simulink model "NonisothermalCSTR_closedLoop"  (R2024a)
settings: Solver=ode23s  StartTime=0.0  StopTime=3600*4  RelTol=1e-3
undefined symbols (not defined in the file): u_simulate
libraries: slpidlib x3
settings Model: Creator=tmlouw  LastModifiedBy=tmlouw

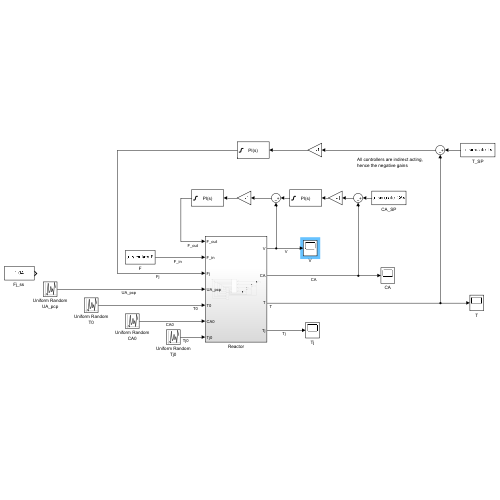
[thumbnail: Simulink's stored preview of the top-level diagram]
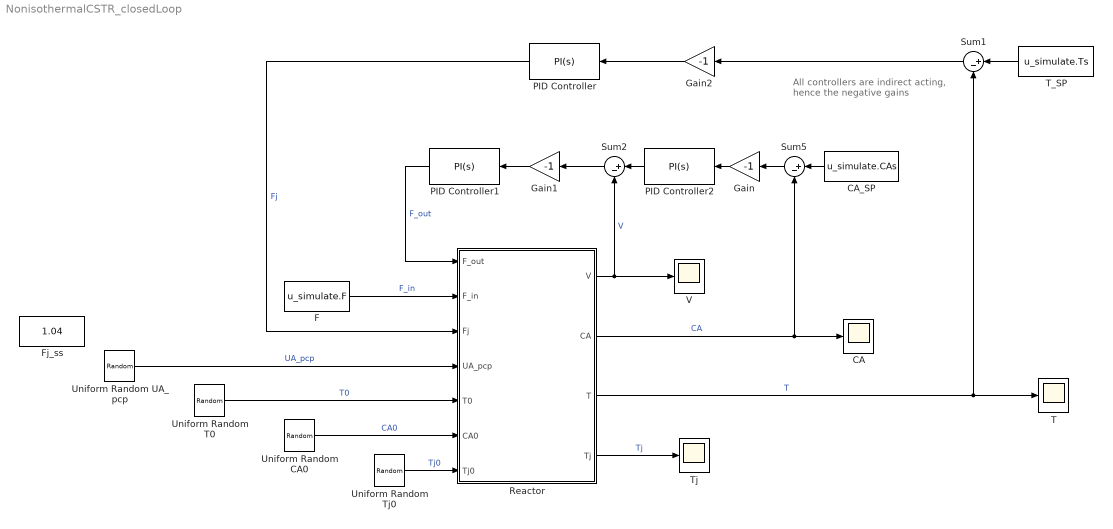
== system NonisothermalCSTR_closedLoop ==
  note: All controllers are indirect acting, hence the negative gains
  CA : Scope
  CA_SP : Constant  Value=u_simulate.CAs
  F : Constant  Value=u_simulate.F
  "Fj_ss " : Constant  Value=1.04
  Gain : Gain  Gain=-1
  Gain1 : Gain  Gain=-1
  Gain2 : Gain  Gain=-1
  PID Controller : slpidlib/PID Controller  Controller=PI  Form=Parallel  TimeDomain=Continuous-time  UseExternalTs=off  SampleTime=-1  IntegratorMethod=Forward Euler  FilterMethod=Forward Euler  ControllerParametersSource=internal  P=10  I=0  UseKiTs=off  D=0  UseExternalDerivativeSource=off  N=100  UseFilter=on  TunerSelectOption=Transfer Function Based (PID Tuner App)  InitialConditionSource=internal  InitialConditionForIntegrator=1.04  InitialConditionForFilter=0  DifferentiatorICPrevScaledInput=0  ExternalReset=none  TrackingMode=off  Kt=1  LimitOutput=on  SatLimitsSource=internal  UpperSaturationLimit=5  LowerSaturationLimit=0  LinearizeAsGain=on  AntiWindupMode=clamping  Kb=1  LimitIntegrator=off  UpperIntegratorSaturationLimit=inf  LowerIntegratorSaturationLimit=-inf  POutMin=[]  POutMax=[]  IOutMin=[]  IOutMax=[]  DOutMin=[]  DOutMax=[]  NOutMin=[]  NOutMax=[]  SumOutMin=[]  SumOutMax=[]  SaturationOutMin=[]  SaturationOutMax=[]  PParamMin=[]  PParamMax=[]  IParamMin=[]  IParamMax=[]  DParamMin=[]  DParamMax=[]  NParamMin=[]  NParamMax=[]  KbParamMin=[]  KbParamMax=[]  KtParamMin=[]  KtParamMax=[]  KbOutMin=[]  KbOutMax=[]  KtOutMin=[]  KtOutMax=[]  IntegratorOutMin=[]  IntegratorOutMax=[]  FilterOutMin=[]  FilterOutMax=[]  SumI1OutMin=[]  SumI1OutMax=[]  SumI2OutMin=[]  SumI2OutMax=[]  SumI3OutMin=[]  SumI3OutMax=[]  SumI4OutMin=[]  SumI4OutMax=[]  SumDOutMin=[]  SumDOutMax=[]  DifferentiatorOutMin=[]  DifferentiatorOutMax=[]  FilterDiffOutCoefMin=[]  FilterDiffOutCoefMax=[]  ReciprocalOutMin=[]  ReciprocalOutMax=[]  SumDenOutMin=[]  SumDenOutMax=[]  SumNumOutMin=[]  SumNumOutMax=[]  DivideOutMin=[]  DivideOutMax=[]  UdiffTsProdOutMin=[]  UdiffTsProdOutMax=[]  NTsProdOutMin=[]  NTsProdOutMax=[]  UintegralTsProdOutMin=[]  UintegralTsProdOutMax=[]  UngainTsProdOutMin=[]  UngainTsProdOutMax=[]  ClampingZeroOutDataTypeStr=Inherit: Inherit via back propagation  ClampingZeroOutMin=[]  ClampingZeroOutMax=[]  FilterDenConstantOutDataTypeStr=Inherit: Inherit via back propagation  FilterDenConstantOutMin=[]  FilterDenConstantOutMax=[]  PCopyOutDataTypeStr=Inherit: Inherit via back propagation  PCopyOutMin=[]  PCopyOutMax=[]  NCopyOutDataTypeStr=Inherit: Inherit via back propagation  NCopyOutMin=[]  NCopyOutMax=[]  IntegratorContinuousStateAttributes=''  IntegratorStateMustResolveToSignalObject=off  IntegratorRTWStateStorageClass=Auto  FilterContinuousStateAttributes=''  FilterStateMustResolveToSignalObject=off  FilterRTWStateStorageClass=Auto  ParallelPVariant=InternalParameters  IdealPVariant=Disabled  IVariant=InternalParameters  DVariant=Disabled  IntegratorVariant=Continuous  SatVariant=Enabled  AWVariant=ContClampingParallel  PCopyVariant=Disabled  TRVariant=Disabled  FdbkBlocksVariant=Forward  IdealPFdbkVariant=Disabled  SatFdbkVariant=Disabled  DerivativeFilterVariant=Disabled  NVariant=Disabled  NCopyVariant=Disabled_SignalSpec  FilterICVariant=Disabled  IntegratorICVariant=InternalICs  ExternalResetVariant=Disabled  TRSumVariant=Passthrough  SumFdbkVariant=Disabled  SumVariant=Sum_PI  TsampFilterVariant=InternalTs  TsampNgainVariant=Passthrough  TsampIntegralVariant=Disabled_SignalSpec  ExternalSaturationOutDataTypeStr=Inherit: Same as second input  DerivativeSourceVariant=Disabled
  PID Controller1 : slpidlib/PID Controller  Controller=PI  Form=Parallel  TimeDomain=Continuous-time  UseExternalTs=off  SampleTime=-1  IntegratorMethod=Forward Euler  FilterMethod=Forward Euler  ControllerParametersSource=internal  P=50  I=0  UseKiTs=off  D=0  UseExternalDerivativeSource=off  N=100  UseFilter=on  TunerSelectOption=Transfer Function Based (PID Tuner App)  InitialConditionSource=internal  InitialConditionForIntegrator=u_simulate.F  InitialConditionForFilter=0  DifferentiatorICPrevScaledInput=0  ExternalReset=none  TrackingMode=off  Kt=1  LimitOutput=on  SatLimitsSource=internal  UpperSaturationLimit=0.8  LowerSaturationLimit=0.05  LinearizeAsGain=off  AntiWindupMode=none  Kb=1  LimitIntegrator=off  UpperIntegratorSaturationLimit=inf  LowerIntegratorSaturationLimit=-inf  POutMin=[]  POutMax=[]  IOutMin=[]  IOutMax=[]  DOutMin=[]  DOutMax=[]  NOutMin=[]  NOutMax=[]  SumOutMin=[]  SumOutMax=[]  SaturationOutMin=[]  SaturationOutMax=[]  PParamMin=[]  PParamMax=[]  IParamMin=[]  IParamMax=[]  DParamMin=[]  DParamMax=[]  NParamMin=[]  NParamMax=[]  KbParamMin=[]  KbParamMax=[]  KtParamMin=[]  KtParamMax=[]  KbOutMin=[]  KbOutMax=[]  KtOutMin=[]  KtOutMax=[]  IntegratorOutMin=[]  IntegratorOutMax=[]  FilterOutMin=[]  FilterOutMax=[]  SumI1OutMin=[]  SumI1OutMax=[]  SumI2OutMin=[]  SumI2OutMax=[]  SumI3OutMin=[]  SumI3OutMax=[]  SumI4OutMin=[]  SumI4OutMax=[]  SumDOutMin=[]  SumDOutMax=[]  DifferentiatorOutMin=[]  DifferentiatorOutMax=[]  FilterDiffOutCoefMin=[]  FilterDiffOutCoefMax=[]  ReciprocalOutMin=[]  ReciprocalOutMax=[]  SumDenOutMin=[]  SumDenOutMax=[]  SumNumOutMin=[]  SumNumOutMax=[]  DivideOutMin=[]  DivideOutMax=[]  UdiffTsProdOutMin=[]  UdiffTsProdOutMax=[]  NTsProdOutMin=[]  NTsProdOutMax=[]  UintegralTsProdOutMin=[]  UintegralTsProdOutMax=[]  UngainTsProdOutMin=[]  UngainTsProdOutMax=[]  ClampingZeroOutDataTypeStr=Inherit: Inherit via back propagation  ClampingZeroOutMin=[]  ClampingZeroOutMax=[]  FilterDenConstantOutDataTypeStr=Inherit: Inherit via back propagation  FilterDenConstantOutMin=[]  FilterDenConstantOutMax=[]  PCopyOutDataTypeStr=Inherit: Inherit via back propagation  PCopyOutMin=[]  PCopyOutMax=[]  NCopyOutDataTypeStr=Inherit: Inherit via back propagation  NCopyOutMin=[]  NCopyOutMax=[]  IntegratorContinuousStateAttributes=''  IntegratorStateMustResolveToSignalObject=off  IntegratorRTWStateStorageClass=Auto  FilterContinuousStateAttributes=''  FilterStateMustResolveToSignalObject=off  FilterRTWStateStorageClass=Auto  ParallelPVariant=InternalParameters  IdealPVariant=Disabled  IVariant=InternalParameters  DVariant=Disabled  IntegratorVariant=Continuous  SatVariant=Enabled  AWVariant=Passthrough  PCopyVariant=Disabled  TRVariant=Disabled  FdbkBlocksVariant=Forward  IdealPFdbkVariant=Disabled  SatFdbkVariant=Disabled  DerivativeFilterVariant=Disabled  NVariant=Disabled  NCopyVariant=Disabled_SignalSpec  FilterICVariant=Disabled  IntegratorICVariant=InternalICs  ExternalResetVariant=Disabled  TRSumVariant=Passthrough  SumFdbkVariant=Disabled  SumVariant=Sum_PI  TsampFilterVariant=InternalTs  TsampNgainVariant=Passthrough  TsampIntegralVariant=Disabled_SignalSpec  ExternalSaturationOutDataTypeStr=Inherit: Same as second input  DerivativeSourceVariant=Disabled
  PID Controller2 : slpidlib/PID Controller  Controller=PI  Form=Parallel  TimeDomain=Continuous-time  UseExternalTs=off  SampleTime=-1  IntegratorMethod=Forward Euler  FilterMethod=Forward Euler  ControllerParametersSource=internal  P=1000  I=0  UseKiTs=off  D=0  UseExternalDerivativeSource=off  N=100  UseFilter=on  TunerSelectOption=Transfer Function Based (PID Tuner App)  InitialConditionSource=internal  InitialConditionForIntegrator=u_simulate.V  InitialConditionForFilter=0  DifferentiatorICPrevScaledInput=0  ExternalReset=none  TrackingMode=off  Kt=1  LimitOutput=on  SatLimitsSource=internal  UpperSaturationLimit=500  LowerSaturationLimit=100  LinearizeAsGain=on  AntiWindupMode=clamping  Kb=1  LimitIntegrator=off  UpperIntegratorSaturationLimit=inf  LowerIntegratorSaturationLimit=-inf  POutMin=[]  POutMax=[]  IOutMin=[]  IOutMax=[]  DOutMin=[]  DOutMax=[]  NOutMin=[]  NOutMax=[]  SumOutMin=[]  SumOutMax=[]  SaturationOutMin=[]  SaturationOutMax=[]  PParamMin=[]  PParamMax=[]  IParamMin=[]  IParamMax=[]  DParamMin=[]  DParamMax=[]  NParamMin=[]  NParamMax=[]  KbParamMin=[]  KbParamMax=[]  KtParamMin=[]  KtParamMax=[]  KbOutMin=[]  KbOutMax=[]  KtOutMin=[]  KtOutMax=[]  IntegratorOutMin=[]  IntegratorOutMax=[]  FilterOutMin=[]  FilterOutMax=[]  SumI1OutMin=[]  SumI1OutMax=[]  SumI2OutMin=[]  SumI2OutMax=[]  SumI3OutMin=[]  SumI3OutMax=[]  SumI4OutMin=[]  SumI4OutMax=[]  SumDOutMin=[]  SumDOutMax=[]  DifferentiatorOutMin=[]  DifferentiatorOutMax=[]  FilterDiffOutCoefMin=[]  FilterDiffOutCoefMax=[]  ReciprocalOutMin=[]  ReciprocalOutMax=[]  SumDenOutMin=[]  SumDenOutMax=[]  SumNumOutMin=[]  SumNumOutMax=[]  DivideOutMin=[]  DivideOutMax=[]  UdiffTsProdOutMin=[]  UdiffTsProdOutMax=[]  NTsProdOutMin=[]  NTsProdOutMax=[]  UintegralTsProdOutMin=[]  UintegralTsProdOutMax=[]  UngainTsProdOutMin=[]  UngainTsProdOutMax=[]  ClampingZeroOutDataTypeStr=Inherit: Inherit via back propagation  ClampingZeroOutMin=[]  ClampingZeroOutMax=[]  FilterDenConstantOutDataTypeStr=Inherit: Inherit via back propagation  FilterDenConstantOutMin=[]  FilterDenConstantOutMax=[]  PCopyOutDataTypeStr=Inherit: Inherit via back propagation  PCopyOutMin=[]  PCopyOutMax=[]  NCopyOutDataTypeStr=Inherit: Inherit via back propagation  NCopyOutMin=[]  NCopyOutMax=[]  IntegratorContinuousStateAttributes=''  IntegratorStateMustResolveToSignalObject=off  IntegratorRTWStateStorageClass=Auto  FilterContinuousStateAttributes=''  FilterStateMustResolveToSignalObject=off  FilterRTWStateStorageClass=Auto  ParallelPVariant=InternalParameters  IdealPVariant=Disabled  IVariant=InternalParameters  DVariant=Disabled  IntegratorVariant=Continuous  SatVariant=Enabled  AWVariant=ContClampingParallel  PCopyVariant=Disabled  TRVariant=Disabled  FdbkBlocksVariant=Forward  IdealPFdbkVariant=Disabled  SatFdbkVariant=Disabled  DerivativeFilterVariant=Disabled  NVariant=Disabled  NCopyVariant=Disabled_SignalSpec  FilterICVariant=Disabled  IntegratorICVariant=InternalICs  ExternalResetVariant=Disabled  TRSumVariant=Passthrough  SumFdbkVariant=Disabled  SumVariant=Sum_PI  TsampFilterVariant=InternalTs  TsampNgainVariant=Passthrough  TsampIntegralVariant=Disabled_SignalSpec  ExternalSaturationOutDataTypeStr=Inherit: Same as second input  DerivativeSourceVariant=Disabled
  Reactor : Subsystem
  Sum1 : Sum  Inputs=|+-
  Sum2 : Sum  Inputs=|+-
  Sum5 : Sum  Inputs=|+-
  T : Scope
  T_SP : Constant  Value=u_simulate.Ts
  Tj : Scope
  Uniform Random CA0 : UniformRandomNumber  Minimum=19  Maximum=21  Seed=1  SampleTime=200
  Uniform Random T0 : UniformRandomNumber  Minimum=295  Maximum=305  Seed=2  SampleTime=200
  Uniform Random Tj0 : UniformRandomNumber  Minimum=278  Maximum=288  SampleTime=200
  Uniform Random UA_pcp : UniformRandomNumber  Minimum=0.33  Maximum=0.37  Seed=3  SampleTime=500
  V : Scope
  wires:
  Uniform Random UA_pcp/1 -> Reactor/4(UA_pcp)  "UA_pcp"
  Uniform Random T0/1 -> Reactor/5(T0)  "T0"
  Uniform Random CA0/1 -> Reactor/6(CA0)  "CA0"
  Reactor/1(V) -> V/1, Sum2/2  "V"
  Reactor/2(CA) -> Sum5/2, CA/1  "CA"
  Reactor/3(T) -> Sum1/2, T/1  "T"
  Reactor/4(Tj) -> Tj/1  "Tj"
  F/1 -> Reactor/2(F_in)  "F_in"
  PID Controller/1 -> Reactor/3(Fj)  "Fj"
  T_SP/1 -> Sum1/1
  Sum1/1 -> Gain2/1
  Sum2/1 -> Gain1/1
  PID Controller1/1 -> Reactor/1(F_out)  "F_out"
  PID Controller2/1 -> Sum2/1
  CA_SP/1 -> Sum5/1
  Sum5/1 -> Gain/1
  Uniform Random Tj0/1 -> Reactor/7(Tj0)  "Tj0"
  Gain/1 -> PID Controller2/1
  Gain1/1 -> PID Controller1/1
  Gain2/1 -> PID Controller/1

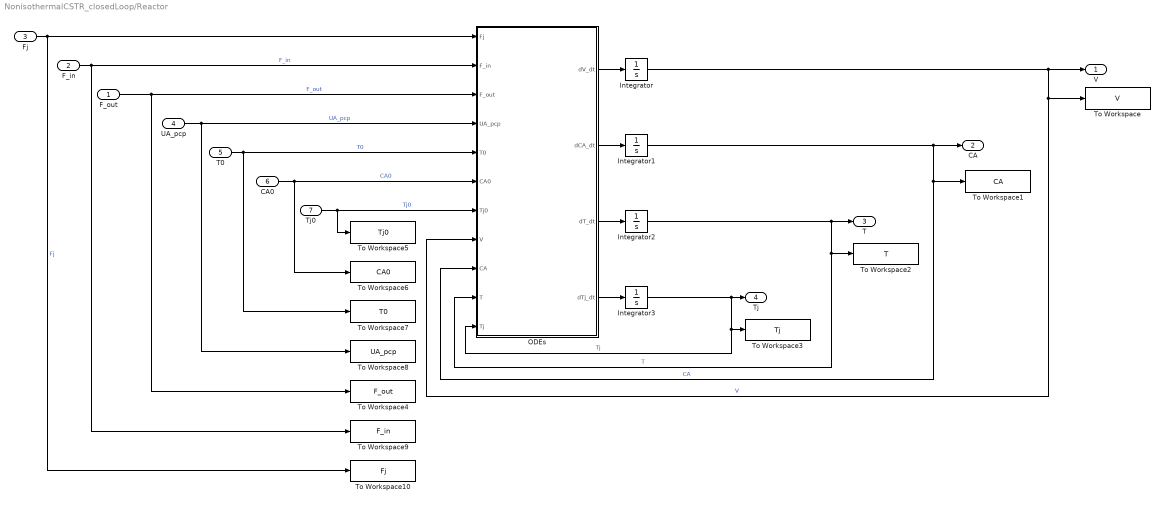
== system NonisothermalCSTR_closedLoop/Reactor ==
  F_out : Inport
  F_in : Inport  Port=2
  Fj : Inport  Port=3
  UA_pcp : Inport  Port=4
  T0 : Inport  Port=5
  CA0 : Inport  Port=6
  Tj0 : Inport  Port=7
  Integrator : Integrator  InitialCondition=u_simulate.V
  Integrator1 : Integrator  InitialCondition=u_simulate.CAs
  Integrator2 : Integrator  InitialCondition=u_simulate.Ts
  Integrator3 : Integrator  InitialCondition=u_simulate.Tjs
  ODEs : MATLAB Function  TreatAsAtomicUnit=on
  To Workspace : ToWorkspace  VariableName=V  SampleTime=1
  To Workspace1 : ToWorkspace  VariableName=CA  SampleTime=1
  To Workspace10 : ToWorkspace  VariableName=Fj  SampleTime=1
  To Workspace2 : ToWorkspace  VariableName=T  SampleTime=1
  To Workspace3 : ToWorkspace  VariableName=Tj  SampleTime=1
  To Workspace4 : ToWorkspace  VariableName=F_out  SampleTime=1
  To Workspace5 : ToWorkspace  VariableName=Tj0  SampleTime=1
  To Workspace6 : ToWorkspace  VariableName=CA0  SampleTime=1
  To Workspace7 : ToWorkspace  VariableName=T0  SampleTime=1
  To Workspace8 : ToWorkspace  VariableName=UA_pcp  SampleTime=1
  To Workspace9 : ToWorkspace  VariableName=F_in  SampleTime=1
  V : Outport
  CA : Outport  Port=2
  T : Outport  Port=3
  Tj : Outport  Port=4
  wires:
  Integrator3/1 -> ODEs/11(Tj), To Workspace3/1, Tj/1  "Tj"
  Integrator2/1 -> T/1, To Workspace2/1, ODEs/10(T)  "T"
  ODEs/1(dV_dt) -> Integrator/1
  ODEs/2(dCA_dt) -> Integrator1/1
  Integrator/1 -> V/1, To Workspace/1, ODEs/8(V)  "V"
  ODEs/3(dT_dt) -> Integrator2/1
  ODEs/4(dTj_dt) -> Integrator3/1
  F_in/1 -> To Workspace9/1, ODEs/2(F_in)  "F_in"
  T0/1 -> ODEs/5(T0), To Workspace7/1  "T0"
  UA_pcp/1 -> To Workspace8/1, ODEs/4(UA_pcp)  "UA_pcp"
  CA0/1 -> To Workspace6/1, ODEs/6(CA0)  "CA0"
  F_out/1 -> ODEs/3(F_out), To Workspace4/1  "F_out"
  Tj0/1 -> ODEs/7(Tj0), To Workspace5/1  "Tj0"
  Integrator1/1 -> CA/1, To Workspace1/1, ODEs/9(CA)  "CA"
  Fj/1 -> To Workspace10/1, ODEs/1(Fj)  "Fj"

== matlab function NonisothermalCSTR_closedLoop/Reactor/ODEs ==
  data: Fj input; F_in input; F_out input; UA_pcp input; T0 input; CA0 input; Tj0 input; V input; CA input; T input; Tj input; dV_dt output; dCA_dt output; dT_dt output; dTj_dt output
function [dV_dt, dCA_dt, dT_dt, dTj_dt] = ODEs(Fj, F_in, F_out, UA_pcp, T0, CA0, Tj0, V, CA, T, Tj)

% Process parameters
dH_pcp = 5; % K.L/mol, heat of reaction divided by molar heat capacity
E_R = 6000; % K, activation energy divided by universal gas constant
k0 = 2.7e5; % 1/s, pre-exponential rate coefficient
Vj = 10;    % L, cooling jacket volume

rxn = k0*CA*exp(-E_R / T);

dV_dt = F_in - F_out;
dCA_dt = F_in/V*(CA0 - CA) - rxn;
dT_dt = F_in/V*(T0 - T) + dH_pcp*rxn - UA_pcp/V*(T - Tj);
dTj_dt = Fj/Vj*(Tj0 - Tj) + UA_pcp/Vj*(T - Tj);
